simulink model "METI_TRAMI_Thermal_ver01_Jmaab_2018b_Intg"  (R2018b)
settings: Solver=ode8  StartTime=0  StopTime=end_time  FixedStep=sampling_time  RelTol=1e-3
PreLoadFcn:
  | METI_TRAMI_Thermal_ver01_Jmaab_PreLoad;
values from neighbouring files (symbols this model uses):
  degC2K = 273.15    [METI_TRAMI_Thermal_ver01_Jmaab_PreLoad.m]    (also in init_setting_METI.m)
  K2degC = -273.15    [METI_TRAMI_Thermal_ver01_Jmaab_PreLoad.m]    (also in init_setting_METI.m)
undefined symbols (not defined in the file or in its folder): ACC_D_Gain, ACC_I_Gain, ACC_P_Gain, ALT_CNT_ALT_OFF_RPM_HYS_rpm, ALT_CNT_ALT_ON_RPM_HYS_rpm, ALT_CNT_Alter_V_BASE_V, ALT_CNT_Alter_V_Kaisei_V, ALT_CNT_flag_disable_kaisei, ALT_CNT_V_Battely_Kudo_V, ALT_PNT_ALT_GDCurrent_A, ALT_PNT_ALT_GDVolt_V, ALT_PNT_Alter_limit_Current_V_table, ALT_PNT_Alter_limit_Current_V_table_x_rpm, ALT_PNT_Alter_trq_Nm_map, ALT_PNT_Alter_trq_Nm_map_x_rpm, ALT_PNT_Alter_trq_Nm_map_y_Current_A, ALT_PNT_Alter_trq_Nm_map_z_Volt_tgt_V, ALT_PNT_eta_pulley_alt, ALT_PNT_Gain_Alt_v_del, ALT_PNT_ratio_pulley_alt, ALT_PNT_Tau_Alternator_V_tgt_s, ALT_PNT_trq_alter_output_LL_Nm, BK_PNT_Pow_UL, BK_PNT_Tau_brake, Brk_LL, Brk_PGain, Brk_UL, BT_PNT_Lo_Capa_lo_batt_F, BT_PNT_Lo_ocv_SOC_lo_batt_OCV_V_table, BT_PNT_Lo_ocv_SOC_lo_batt_OCV_V_table_x_SOC, BT_PNT_Lo_R_lo_batt_ohm, BT_PNT_Lo_SOC_MAX_lo_batt, BT_PNT_Lo_SOC_MIN_lo_batt, BT_PNT_Lo_SOC_START_lo_batt, BT_PNT_Lo_V_start_ocv, DF_PNT_DF_gear, DF_PNT_DFBlock2DFAir_Heat_Resi_KpW, DF_PNT_DFBlock_Heat_Capa_JpK, DF_PNT_DFBlock_Temp_ini_degC, DF_PNT_DFOil2DFBlock_Heat_Resi_KpW, DF_PNT_DFOil_Heat_Capa_JpK, DF_PNT_DFOil_Temp_ini_degC, DF_PNT_Driveshaft_damper, DF_PNT_Driveshaft_delta_radps_LL, DF_PNT_Driveshaft_delta_radps_UL, DF_PNT_Driveshaft_spring, DF_PNT_eta_DF, DF_PNT_Outtemp_degC, DF_PNT_TMBlock2DFBlock_Heat_Resi_KpW, Driver_Brake_Const1, Driver_Brake_Const3, Driver_Brake_Switch_Const2, Driver_Brk_sh, drivmode_ACC, drivmode_CONST, drivmode_GensokuKaisei, drivmode_GensokuRikko, drivmode_STOP, EL_PNT_R_bodyelec_lo_ohm, ENG_CNT_acc_idlestop ... (+139)
libraries: METI_Lib_vehicle_model x33, simulink x7, AZAPA_Lib_vehicle_model x1
(part 2 of 4)

== system METI_TRAMI_Thermal_ver01_Jmaab_2018b_Intg/Vehicle/ALT_PNT/pulley_slave ==
  note: プーリー比
  note: プーリー効率
  w_ENG_PNT_radps : Inport
  trq_slavepulley12 : Inport  Port=2
  P_cal : AZAPA_Lib_vehicle_model/P_cal  Commented=on  Type_energy=並進運動  Type_output_energy=出力  Power_name=Po_  t_Workspace_Name=MOTOR_MECK  P_VariableName=Po_MOTOR_MECK  Across_VariableName=v_MOTOR_MECK  Throgh_VariableName=F_MOTOR_MECK
  Product : Product  RndMeth=Zero
  Product1 : Product  RndMeth=Zero
  eta_cal2 : METI_Lib_vehicle_model/eta_cal2  SystemSampleTime=-1
  eta_pulley : Constant  Value=ALT_PNT_eta_pulley_alt
  ratio_pulley : Constant  Value=ALT_PNT_ratio_pulley_alt
  trq_slavepulley11 : Outport
  w_slavepulley12 : Outport  Port=2
  tag scope: tScope_pulley1Loss=global
  wires:
  eta_cal2/1 -> P_cal/2
  P_cal/1 -> [tScope_pulley1Loss]
  w_ENG_PNT_radps/1 -> P_cal/1, Product1/1
  eta_cal2/2 -> trq_slavepulley11/1
  trq_slavepulley12/1 -> Product/2
  eta_pulley/1 -> eta_cal2/1
  Product1/1 -> w_slavepulley12/1
  ratio_pulley/1 -> Product/1, Product1/2
  Product/1 -> eta_cal2/2

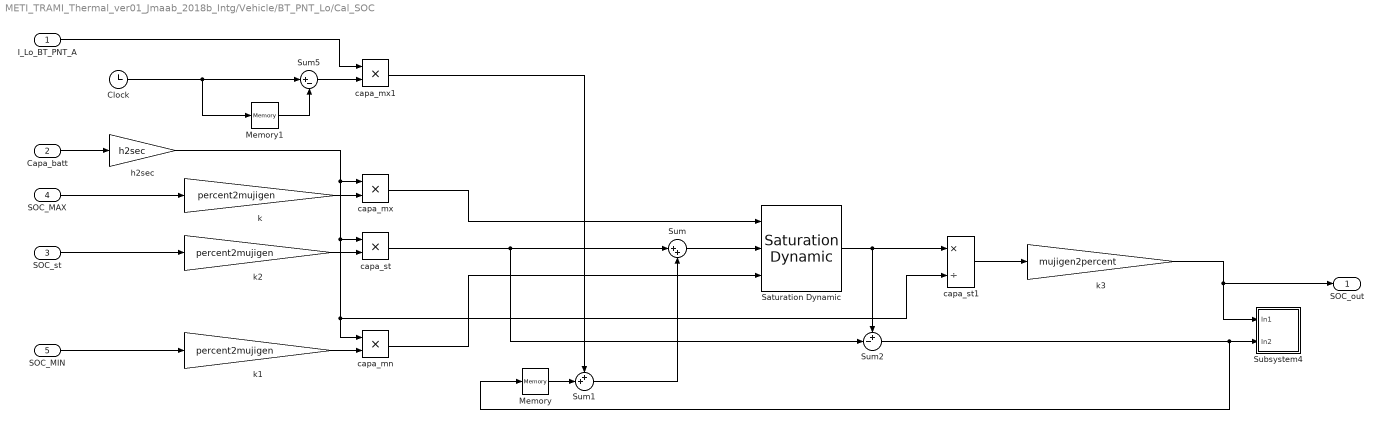
== system METI_TRAMI_Thermal_ver01_Jmaab_2018b_Intg/Vehicle/BT_PNT_Lo/Cal_SOC ==
  I_Lo_BT_PNT_A : Inport
  Capa_batt : Inport  Port=2
  SOC_st : Inport  Port=3
  SOC_MAX : Inport  Port=4
  SOC_MIN : Inport  Port=5
  Clock : Clock
  Memory : Memory
  Memory1 : Memory
  Saturation Dynamic : simulink/Discontinuities/Saturation Dynamic  OutMin=[]  OutMax=[]  OutDataTypeStr=Inherit: Same as second input  OutDataType=fixdt(1, 16)  OutScaling=2^-10  DoSatur=off
  Subsystem4 : Subsystem  mask{SOC=SOC_LoBat, VariableName=Asec_LoBat}
      mask prompts: SOC "バッテリSOC"; VariableName "バッテリ容量変化量(Asec)"
  Sum : Sum  Inputs=|++
  Sum1 : Sum  Inputs=++|
  Sum2 : Sum  Inputs=+-|
  Sum5 : Sum  Inputs=|+-
  capa_mn : Product  RndMeth=Zero
  capa_mx : Product  RndMeth=Zero
  capa_mx1 : Product  RndMeth=Zero
  capa_st : Product  RndMeth=Zero
  capa_st1 : Product  Inputs=*/  RndMeth=Zero
  h2sec : Gain  Gain=h2sec
  k : Gain  Gain=percent2mujigen
  k1 : Gain  Gain=percent2mujigen
  k2 : Gain  Gain=percent2mujigen
  k3 : Gain  Gain=mujigen2percent
  SOC_out : Outport
  wires:
  Sum5/1 -> capa_mx1/2
  Memory1/1 -> Sum5/2
  Sum/1 -> Saturation Dynamic/2
  Clock/1 -> Sum5/1, Memory1/1
  capa_mx1/1 -> Sum1/1
  k3/1 -> Subsystem4/1(In1), SOC_out/1
  Sum1/1 -> Sum/2
  Memory/1 -> Sum1/2
  k2/1 -> capa_st/2
  k1/1 -> capa_mn/2
  k/1 -> capa_mx/2
  capa_st/1 -> Sum2/2, Sum/1
  Saturation Dynamic/1 -> Sum2/1, capa_st1/1
  capa_mx/1 -> Saturation Dynamic/1
  capa_mn/1 -> Saturation Dynamic/3
  capa_st1/1 -> k3/1
  h2sec/1 -> capa_mn/1, capa_st1/2, capa_st/1, capa_mx/1
  SOC_MIN/1 -> k1/1
  SOC_MAX/1 -> k/1
  SOC_st/1 -> k2/1
  Capa_batt/1 -> h2sec/1
  I_Lo_BT_PNT_A/1 -> capa_mx1/1
  Sum2/1 -> Memory/1, Subsystem4/2(In2)

== system METI_TRAMI_Thermal_ver01_Jmaab_2018b_Intg/Vehicle/BT_PNT_Lo/Subsystem ==
  I_BT_PNT_Lo_A : Inport
  Divide : Product
  Resistivity : Constant  Value=BT_PNT_Lo_R_lo_batt_ohm
  Sum : Sum  Inputs=|++
  Transfer Fcn : TransferFcn  Numerator=[0.01]  Denominator=[0.1 1]
  V_BT_PNT_Lo_V : Outport
  wires:
  Resistivity/1 -> Divide/2
  Divide/1 -> Sum/1
  I_BT_PNT_Lo_A/1 -> Divide/1, Transfer Fcn/1
  Sum/1 -> V_BT_PNT_Lo_V/1
  Transfer Fcn/1 -> Sum/2

== system METI_TRAMI_Thermal_ver01_Jmaab_2018b_Intg/Vehicle/CNT/ALT_CNT ==
  sensor_BT_PNT_Lo_BUS : Inport
  ALT_Ctrl : Subsystem
  Bus Creator6 : BusCreator  Inputs=1
  Bus Selector1 : BusSelector  OutputSignals=flag_fuelcut,flag_IdleStop,n_eng_rpm
  Bus Selector9 : BusSelector  OutputSignals=SOC_BT_PNT_Lo_PCT
  ALT_CNT_out : Outport
  wires:
  [ALT_CNT_CAN_Rx] -> Bus Selector1/1
  Bus Selector1/1 -> ALT_Ctrl/2(flag_fuelcut)  "<flag_fuelcut>"
  Bus Selector1/2 -> ALT_Ctrl/3(flag_IdleStop)  "<flag_IdleStop>"
  Bus Selector1/3 -> ALT_Ctrl/4(n_eng_rpm)  "<n_eng_rpm>"
  ALT_Ctrl/1(target_volt_ALT_V) -> Bus Creator6/1
  sensor_BT_PNT_Lo_BUS/1 -> Bus Selector9/1
  Bus Selector9/1 -> ALT_Ctrl/1(SOC_BT_PNT_Lo_PCT)  "<SOC_BT_PNT_Lo_PCT>"
  Bus Creator6/1 -> ALT_CNT_out/1  "ALT_CNT_out"

== system METI_TRAMI_Thermal_ver01_Jmaab_2018b_Intg/Vehicle/CNT/BK_CNT ==
  Driver_Input : Inport
  sensor_VL_PNT_BUS : Inport  Port=2
  sensor_BK_PNT : Inport  Port=3
  BK_Ctrl : Subsystem
  Bus Creator1 : BusCreator  Inputs=1
  Bus Creator2 : BusCreator  Inputs=2
  Bus Selector1 : BusSelector  OutputSignals=trq_BK_PNT_Nm
  Bus Selector12 : BusSelector  OutputSignals=v_VL_PNT_kmph
  Bus Selector4 : BusSelector  OutputSignals=open_brake_per
  BK_CNT_out : Outport
  tag scope: BK_CNT_CAN_Tx=scoped
  wires:
  BK_Ctrl/2(v_VL_PNT_kmph) -> Bus Creator2/1
  Bus Selector12/1 -> BK_Ctrl/2(v_VL_PNT_kmph_in)  "<v_VL_PNT_kmph>"
  sensor_VL_PNT_BUS/1 -> Bus Selector12/1
  BK_Ctrl/3(trq_BK_PNT_Nm) -> Bus Creator2/2
  Bus Creator2/1 -> [BK_CNT_CAN_Tx]  "BK_CNT_CAN_Tx"
  Bus Selector1/1 -> BK_Ctrl/3(trq_BK_PNT_Nm_in)  "<trq_BK_PNT_Nm>"
  sensor_BK_PNT/1 -> Bus Selector1/1
  Bus Creator1/1 -> BK_CNT_out/1  "BK_CNT_out"
  Bus Selector4/1 -> BK_Ctrl/1(open_brake_per_in)  "<open_brake_per>"
  Driver_Input/1 -> Bus Selector4/1
  BK_Ctrl/1(open_brake_per) -> Bus Creator1/1

== system METI_TRAMI_Thermal_ver01_Jmaab_2018b_Intg/Vehicle/CNT/CAN ==
  note: CAN Bus Model
  ALT_CNT : Subsystem
  BK_CNT : Subsystem
  ENG_CNT : Subsystem
  Pwtr_CAN : Subsystem
  TM_CNT : Subsystem
  wires:
  Pwtr_CAN/1(Pwtr_CAN) -> BK_CNT/1(Pwtr_CAN), ALT_CNT/1(Pwtr_CAN), TM_CNT/1(Pwtr_CAN), ENG_CNT/1(Pwtr_CAN)
  ENG_CNT/1(ENG_CNT_CAN_Tx) -> Pwtr_CAN/1(ENG_CNT_CAN_Tx)
  TM_CNT/1(TM_CNT_CAN_Tx) -> Pwtr_CAN/2(TM_CNT_CAN_Tx)
  BK_CNT/1(BK_CNT_CAN_Tx) -> Pwtr_CAN/3(BK_CNT_CAN_Tx)

== system METI_TRAMI_Thermal_ver01_Jmaab_2018b_Intg/Vehicle/CNT/ENG_CNT ==
  Driver_Input : Inport
  sensor_ENG_PNT : Inport  Port=2
  Bus Creator : BusCreator  Inputs=6
  Bus Creator1 : BusCreator  Inputs=10
  Bus Selector1 : BusSelector  OutputSignals=v_VL_PNT_kmph,flag_Lockup
  Bus Selector13 : BusSelector  OutputSignals=n_eng_rpm,fuel_consumption,T_ENGTH_PNT_Coolant_degC
  Bus Selector14 : BusSelector  OutputSignals=open_accel_per,open_brake_per
  ENG_Cntrl : Subsystem
  ENG_CNT_out : Outport
  tag scope: ENG_CNT_CAN_Tx=scoped
  wires:
  ENG_Cntrl/11(IdleSpeed_Target) -> Bus Creator/5
  Bus Selector1/1 -> ENG_Cntrl/6(v_VL_PNT_kmph)  "<v_VL_PNT_kmph>"
  Bus Selector13/3 -> ENG_Cntrl/5(T_ENGTH_PNT_Coolant_degC), Bus Creator/6  "<T_ENGTH_PNT_Coolant_degC>"
  Bus Selector13/2 -> ENG_Cntrl/4(fuel_consumption)  "<fuel_consumption>"
  ENG_Cntrl/10(V_ENG_CNT_RDFan_V) -> Bus Creator1/10
  ENG_Cntrl/9(V_ENG_CNT_WP_V) -> Bus Creator1/9
  ENG_Cntrl/8(K_Fuel) -> Bus Creator1/8
  Bus Selector1/2 -> ENG_Cntrl/7(flag_Lockup)  "<flag_Lockup>"
  [ENG_CNT_CAN_Rx] -> Bus Selector1/1
  Bus Selector14/2 -> ENG_Cntrl/2(open_brake_per)  "<open_brake_per>"
  Bus Selector14/1 -> ENG_Cntrl/1(open_accel_per)  "<open_accel_per>"
  Driver_Input/1 -> Bus Selector14/1
  Bus Selector13/1 -> ENG_Cntrl/3(sens_ENG_PNT)  "<n_eng_rpm>"
  sensor_ENG_PNT/1 -> Bus Selector13/1
  Bus Creator1/1 -> ENG_CNT_out/1  "ENG_CNT_out"
  ENG_Cntrl/7(flag_ON_Starter) -> Bus Creator1/7
  ENG_Cntrl/6(n_eng_rpm) -> Bus Creator1/6, Bus Creator/4
  ENG_Cntrl/5(timing_ignition) -> Bus Creator1/5
  ENG_Cntrl/4(fuel_ratio) -> Bus Creator1/4
  ENG_Cntrl/3(flag_fuelcut) -> Bus Creator1/3, Bus Creator/3
  ENG_Cntrl/2(flag_IdleStop) -> Bus Creator1/2, Bus Creator/2
  ENG_Cntrl/1(open_throttle_per) -> Bus Creator1/1, Bus Creator/1
  Bus Creator/1 -> [ENG_CNT_CAN_Tx]  "ENG_CNT_CAN_Tx"

== system METI_TRAMI_Thermal_ver01_Jmaab_2018b_Intg/Vehicle/CNT/TM_CNT ==
  sensor_TM_PNT : Inport
  Rate Transition : RateTransition  Deterministic=off
      settings: AttributesFormatString=|
      | <Integrity = %<Integrity>>
      | <Deterministic = %<Deterministic>>
  Rate Transition1 : RateTransition  Deterministic=off
      settings: AttributesFormatString=|
      | <Integrity = %<Integrity>>
      | <Deterministic = %<Deterministic>>
  Rate Transition2 : RateTransition  Deterministic=off
      settings: AttributesFormatString=|
      | <Integrity = %<Integrity>>
      | <Deterministic = %<Deterministic>>
  TM_CNT : Subsystem  Variant=on  VariantControl=Variant1
  TM_CNT_out : Outport
  tag scope: TM_CNT_CAN_Tx=scoped, TM_CNT_Info=global
  wires:
  sensor_TM_PNT/1 -> Rate Transition/1
  [TM_CNT_CAN_Rx] -> Rate Transition1/1
  Rate Transition2/1 -> TM_CNT_out/1  "TM_CNT_out"
  Rate Transition/1 -> TM_CNT/1("sensor_TM_PNT ")
  Rate Transition1/1 -> TM_CNT/2("TM_CNT_CAN_Rx ")
  TM_CNT/1(" TM_CNT_out") -> Rate Transition2/1
  TM_CNT/2(" TM_CNT_CAN_Tx") -> [TM_CNT_CAN_Tx]
  TM_CNT/3(" TM_CNT_Info") -> [TM_CNT_Info]

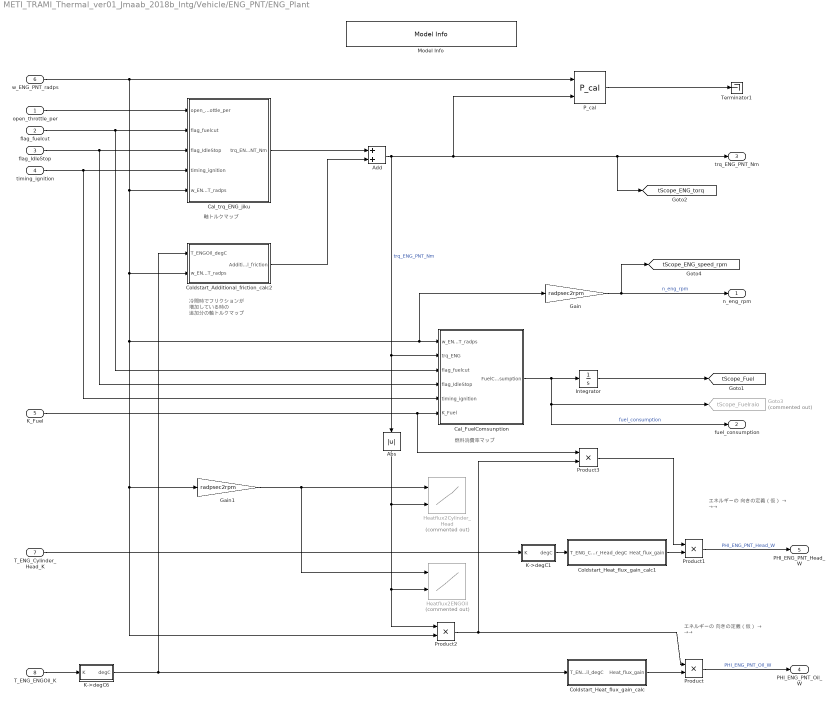
== system METI_TRAMI_Thermal_ver01_Jmaab_2018b_Intg/Vehicle/ENG_PNT/ENG_Plant ==
  note: 軸トルクマップ
  note: 燃料消費率マップ
  note: 冷間時でフリクションが
      | 増加している時の
      | 追加分の軸トルクマップ
  note: エネルギーの
      | 向きの定義（仮）
      | → →→
  note: エネルギーの
      | 向きの定義（仮）
      | → →→
  open_throttle_per : Inport
  flag_fuelcut : Inport  Port=2
  flag_IdleStop : Inport  Port=3
  timing_ignition : Inport  Port=4
  K_Fuel : Inport  Port=5
  w_ENG_PNT_radps : Inport  Port=6
  T_ENG_Cylinder_Head_K : Inport  Port=7
  T_ENG_ENGOil_K : Inport  Port=8
  Abs : Abs
  Add : Sum
  Cal_FuelComsunption : Subsystem
  Cal_trq_ENG_jiku : Subsystem
  Coldstart_Additional_friction_calc2 : Subsystem
  Coldstart_Heat_flux_gain_calc : Subsystem
  Coldstart_Heat_flux_gain_calc1 : Subsystem
  Gain : Gain  Gain=radpsec2rpm
  Gain1 : Gain  Gain=radpsec2rpm
  Goto3 : Goto  Commented=on  GotoTag=tScope_Fuelraio  TagVisibility=global
  Heatflux2Cylinder_Head : Lookup_n-D  Commented=on  BreakpointsForDimension1=ENG_PNT_Heatflux2Cylinder_Head_W_x_rpm  BreakpointsForDimension2=ENG_PNT_Heatflux2Cylinder_Head_W_y_trq  Table=ENG_PNT_Heatflux2Cylinder_Head_W  InternalRulePriority=Speed  RndMeth=Simplest  InputSameDT=on
  Heatflux2ENGOil : Lookup_n-D  Commented=on  BreakpointsForDimension1=ENG_PNT_Heatflux2ENGOil_W_x_rpm  BreakpointsForDimension2=ENG_PNT_Heatflux2ENGOil_W_y_trq  Table=ENG_PNT_Heatflux2ENGOil_W  InternalRulePriority=Speed  RndMeth=Simplest  InputSameDT=on
  Integrator : Integrator
  K->degC1 : Subsystem
  K->degC6 : Subsystem
  Model Info : simulink/Model-Wide Utilities/Model Info  Frame=on  DisplayStringWithTags=【注記】 ・エンジンモデルはトルク出力動作させる側が正  HorizontalTextAlignment=Left  LeftAlignmentValue=0.02
  P_cal : METI_Lib_vehicle_model/P_cal  Type_energy=回転運動  Type_output_energy=出力  Power_name=Po_  t_Workspace_Name=ENG_PNT_MECK  P_VariableName=Po_ENG_PNT_MECK  Across_VariableName=w_ENG_PNT_MECK  Throgh_VariableName=tq_ENG_PNT_MECK
  Product{,1..3} (4 alike) : Product
  Terminator1 : Terminator
  n_eng_rpm : Outport
  fuel_consumption : Outport  Port=2
  trq_ENG_PNT_Nm : Outport  Port=3
  PHI_ENG_PNT_Oil_W : Outport  Port=4
  PHI_ENG_PNT_Head_W : Outport  Port=5
  tag scope: tScope_ENG_speed_rpm=global, tScope_ENG_torq=global, tScope_Fuel=global
  wires:
  Cal_FuelComsunption/1(FuelConsumption) -> fuel_consumption/1, Goto3/1, Integrator/1  "fuel_consumption"
  Integrator/1 -> [tScope_Fuel]
  w_ENG_PNT_radps/1 -> P_cal/1, Coldstart_Additional_friction_calc2/2(w_ENG_PNT_radps), Gain1/1, Product2/2, Gain/1, Cal_FuelComsunption/1(w_ENG_PNT_radps), Cal_trq_ENG_jiku/5(w_ENG_PNT_radps)
  P_cal/1 -> Terminator1/1
  flag_fuelcut/1 -> Cal_trq_ENG_jiku/2(flag_fuelcut), Cal_FuelComsunption/3(flag_fuelcut)
  flag_IdleStop/1 -> Cal_FuelComsunption/4(flag_IdleStop), Cal_trq_ENG_jiku/3(flag_IdleStop)
  open_throttle_per/1 -> Cal_trq_ENG_jiku/1(open_throttle_per)
  Cal_trq_ENG_jiku/1(trq_ENG_PNT_Nm) -> Add/1
  timing_ignition/1 -> Cal_FuelComsunption/5(timing_ignition), Cal_trq_ENG_jiku/4(timing_ignition)
  Gain/1 -> [tScope_ENG_speed_rpm], n_eng_rpm/1  "n_eng_rpm"
  K->degC6/1(degC) -> Coldstart_Heat_flux_gain_calc/1(T_ENGOil_degC), Coldstart_Additional_friction_calc2/1(T_ENGOil_degC)
  T_ENG_Cylinder_Head_K/1 -> K->degC1/1(K)
  Product1/1 -> PHI_ENG_PNT_Head_W/1  "PHI_ENG_PNT_Head_W"
  Product/1 -> PHI_ENG_PNT_Oil_W/1  "PHI_ENG_PNT_Oil_W"
  Gain1/1 -> Heatflux2ENGOil/1, Heatflux2Cylinder_Head/1
  Coldstart_Heat_flux_gain_calc/1(Heat_flux_gain) -> Product/2
  Product2/1 -> Product/1, Product3/2
  Coldstart_Heat_flux_gain_calc1/1(Heat_flux_gain) -> Product1/2
  Coldstart_Additional_friction_calc2/1(Additional_friction) -> Add/2
  Add/1 -> [tScope_ENG_torq], trq_ENG_PNT_Nm/1, P_cal/2, Cal_FuelComsunption/2(trq_ENG), Abs/1  "trq_ENG_PNT_Nm"
  K_Fuel/1 -> Product3/1, Cal_FuelComsunption/6(K_Fuel)
  Abs/1 -> Product2/1, Heatflux2ENGOil/2, Heatflux2Cylinder_Head/2
  Product3/1 -> Product1/1
  T_ENG_ENGOil_K/1 -> K->degC6/1(K)
  K->degC1/1(degC) -> Coldstart_Heat_flux_gain_calc1/1(T_ENG_Cylinder_Head_degC)

== system METI_TRAMI_Thermal_ver01_Jmaab_2018b_Intg/Vehicle/ENG_PNT/K->degC ==
  K : Inport
  Constant2 : Constant  Value=K2degC
  Sum : Sum  Inputs=++|
  degC : Outport
  wires:
  K/1 -> Sum/2
  Constant2/1 -> Sum/1
  Sum/1 -> degC/1

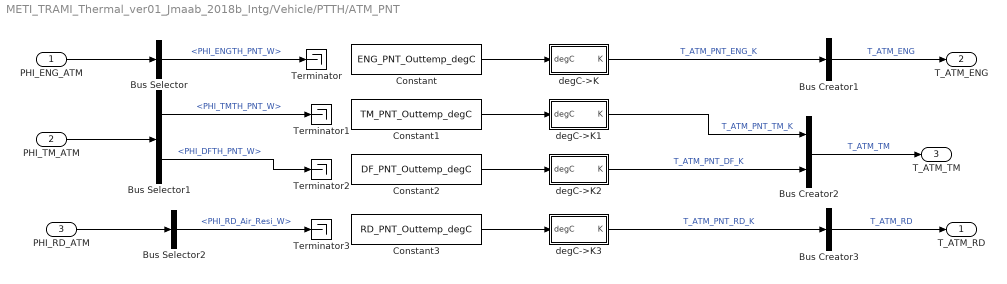
== system METI_TRAMI_Thermal_ver01_Jmaab_2018b_Intg/Vehicle/PTTH/ATM_PNT ==
  PHI_ENG_ATM : Inport
  PHI_TM_ATM : Inport  Port=2
  PHI_RD_ATM : Inport  Port=3
  Bus Creator1 : BusCreator  Inputs=1
  Bus Creator2 : BusCreator  Inputs=2
  Bus Creator3 : BusCreator  Inputs=1
  Bus Selector : BusSelector  OutputSignals=PHI_ENGTH_PNT_W
  Bus Selector1 : BusSelector  OutputSignals=PHI_TMTH_PNT_W,PHI_DFTH_PNT_W
  Bus Selector2 : BusSelector  OutputSignals=PHI_RD_Air_Resi_W
  Constant : Constant  Value=ENG_PNT_Outtemp_degC
  Constant1 : Constant  Value=TM_PNT_Outtemp_degC
  Constant2 : Constant  Value=DF_PNT_Outtemp_degC
  Constant3 : Constant  Value=RD_PNT_Outtemp_degC
  Terminator{,1..3} (4 alike) : Terminator
  degC->K : Subsystem
  degC->K1 : Subsystem
  degC->K2 : Subsystem
  degC->K3 : Subsystem
  T_ATM_RD : Outport
  T_ATM_ENG : Outport  Port=2
  T_ATM_TM : Outport  Port=3
  wires:
  Constant/1 -> degC->K/1(degC)
  Constant1/1 -> degC->K1/1(degC)
  Constant2/1 -> degC->K2/1(degC)
  Constant3/1 -> degC->K3/1(degC)
  Bus Selector1/2 -> Terminator2/1  "<PHI_DFTH_PNT_W>"
  degC->K/1(K) -> Bus Creator1/1  "T_ATM_PNT_ENG_K"
  degC->K1/1(K) -> Bus Creator2/1  "T_ATM_PNT_TM_K"
  degC->K2/1(K) -> Bus Creator2/2  "T_ATM_PNT_DF_K"
  degC->K3/1(K) -> Bus Creator3/1  "T_ATM_PNT_RD_K"
  PHI_ENG_ATM/1 -> Bus Selector/1
  Bus Selector/1 -> Terminator/1  "<PHI_ENGTH_PNT_W>"
  PHI_TM_ATM/1 -> Bus Selector1/1
  Bus Selector1/1 -> Terminator1/1  "<PHI_TMTH_PNT_W>"
  Bus Creator2/1 -> T_ATM_TM/1  "T_ATM_TM"
  Bus Creator1/1 -> T_ATM_ENG/1  "T_ATM_ENG"
  Bus Creator3/1 -> T_ATM_RD/1  "T_ATM_RD"
  PHI_RD_ATM/1 -> Bus Selector2/1
  Bus Selector2/1 -> Terminator3/1  "<PHI_RD_Air_Resi_W>"

== system METI_TRAMI_Thermal_ver01_Jmaab_2018b_Intg/Vehicle/PTTH/DTTH_PNT ==
  T_ENG_TM : Inport
  TM_CNT_out : Inport  Port=2
  PHI_TM_PNT : Inport  Port=3
  v_VL_PNT_mps : Inport  Port=4
  T_RD_TM : Inport  Port=5
  T_ATM_TM : Inport  Port=6
  DTTH_PNT : Subsystem  Variant=on  VariantControl=Variant1
  Memory1 : Memory
  T_TMTH_PNT : Outport
  PHI_TM_ATM : Outport  Port=2
  PHI_TM_RD : Outport  Port=3
  PHI_TM_ENG : Outport  Port=4
  tag scope: TMTH_Info=global
  wires:
  Memory1/1 -> T_TMTH_PNT/1  "T_TMTH_PNT"
  TM_CNT_out/1 -> DTTH_PNT/1("TM_CNT_out ")
  PHI_TM_PNT/1 -> DTTH_PNT/2("PHI_TM_PNT ")
  T_ENG_TM/1 -> DTTH_PNT/3("T_ENG_TM ")
  T_RD_TM/1 -> DTTH_PNT/4("T_RD_TM ")
  T_ATM_TM/1 -> DTTH_PNT/5("T_ATM_TM ")
  v_VL_PNT_mps/1 -> DTTH_PNT/6("v_VL_PNT_mps ")
  DTTH_PNT/1(" T_TMTH_PNT") -> Memory1/1
  DTTH_PNT/2(" PHI_TM_ENG") -> PHI_TM_ENG/1
  DTTH_PNT/3(" PHI_TM_RD") -> PHI_TM_RD/1
  DTTH_PNT/4(" PHI_TM_ATM") -> PHI_TM_ATM/1
  DTTH_PNT/5(" TMTH_Info") -> [TMTH_Info]

== system METI_TRAMI_Thermal_ver01_Jmaab_2018b_Intg/Vehicle/PTTH/ENGTH_PNT ==
  ENG_CNT_out : Inport
  PHI_ENG_PNT : Inport  Port=2
  PHI_RD_ENG : Inport  Port=3
  T_ATM_ENG : Inport  Port=4
  PHI_TM_ENG : Inport  Port=5
  Bus Creator1 : BusCreator  Inputs=3
  Bus Creator2 : BusCreator  Inputs=2
  Bus Creator3 : BusCreator  Inputs=4
  Bus Creator4 : BusCreator  Inputs=1
  Bus Creator5 : BusCreator  Inputs=1
  Bus Selector : BusSelector  OutputSignals=V_ENG_CNT_WP_V
  Bus Selector1 : BusSelector  OutputSignals=PHI_ENG_PNT_Head_W,PHI_ENG_PNT_Oil_W
  Bus Selector2 : BusSelector  OutputSignals=PHI_ENGBlock_Resi2_W,PHI_TM_CVTF_Resi_W
  Bus Selector3 : BusSelector  OutputSignals=T_ATM_PNT_ENG_K
  Bus Selector4 : BusSelector  OutputSignals=PHI_RDTH_PNT_W
  ENGTH : Subsystem
  Signal Specification2 : SignalSpecification
  Signal Specification3 : SignalSpecification
  T_ENGTH_PNT : Outport
  PHI_ENG_ATM : Outport  Port=2
  T_ENG_TM : Outport  Port=3
  T_ENG_RD : Outport  Port=4
  tag scope: ENGTH_Info=global
  wires:
  ENG_CNT_out/1 -> Bus Selector/1
  ENGTH/1(T_ENGTH_PNT_Coolant_K) -> Bus Creator3/4, Bus Creator1/2, Bus Creator2/1, Bus Creator4/1
  ENGTH/2(T_ENG_Block_K) -> Bus Creator3/1, Bus Creator2/2
  ENGTH/3(T_ENGTH_PNT_Oil_K) -> Bus Creator3/2, Signal Specification3/1
  ENGTH/4(T_ENGTH_PNT_Head_K) -> Bus Creator3/3, Signal Specification2/1
  ENGTH/5(PHI_ENGTH_PNT_W) -> Bus Creator5/1
  Bus Selector/1 -> ENGTH/1(V_ENG_CNT_WP_V)  "<V_ENG_CNT_WP_V>"
  PHI_ENG_PNT/1 -> Bus Selector1/1
  Bus Selector1/1 -> ENGTH/3(PHI_ENG_PNT_Head_W)  "<PHI_ENG_PNT_Head_W>"
  Bus Selector1/2 -> ENGTH/4(PHI_ENG_PNT_Oil_W)  "<PHI_ENG_PNT_Oil_W>"
  Bus Creator1/1 -> T_ENGTH_PNT/1  "T_ENGTH_PNT"
  Signal Specification2/1 -> Bus Creator1/1  "T_ENGTH_PNT__Head_K"
  Signal Specification3/1 -> Bus Creator1/3  "T_ENGTH_PNT_Oil_K"
  Bus Creator2/1 -> T_ENG_TM/1  "T_ENG_TM"
  Bus Creator4/1 -> T_ENG_RD/1  "T_ENG_RD"
  Bus Creator5/1 -> PHI_ENG_ATM/1  "PHI_ENG_ATM"
  Bus Creator3/1 -> [ENGTH_Info]  "ENGTH_Info"
  PHI_TM_ENG/1 -> Bus Selector2/1
  Bus Selector2/1 -> ENGTH/2(PHI_ENGBlock_W)  "<PHI_ENGBlock_Resi2_W>"
  Bus Selector2/2 -> ENGTH/6(PHI_TM_CVTF_Resi_W)  "<PHI_TM_CVTF_Resi_W>"
  T_ATM_ENG/1 -> Bus Selector3/1
  PHI_RD_ENG/1 -> Bus Selector4/1
  Bus Selector3/1 -> ENGTH/5(T_ATM_PNT_ENG_K)  "<T_ATM_PNT_ENG_K>"
  Bus Selector4/1 -> ENGTH/7(PHI_ENGCoolant_W1)  "<PHI_RDTH_PNT_W>"

== system METI_TRAMI_Thermal_ver01_Jmaab_2018b_Intg/Vehicle/PTTH/RDTH_PNT ==
  PHI_TM_RD : Inport
  T_ENG_RD : Inport  Port=2
  ENG_CNT_out : Inport  Port=3
  v_VL_PNT_mps : Inport  Port=4
  T_ATM_RD : Inport  Port=5
  Bus Creator : BusCreator  Inputs=1
  Bus Creator1 : BusCreator  Inputs=1
  Bus Creator2 : BusCreator  Inputs=1
  Bus Creator4 : BusCreator  Inputs=2
  Bus Selector : BusSelector  OutputSignals=V_ENG_CNT_RDFan_V
  Bus Selector1 : BusSelector  OutputSignals=T_ENGTH_PNT_Coolant_K
  Bus Selector2 : BusSelector  OutputSignals=T_ATM_PNT_RD_K
  Bus Selector3 : BusSelector  OutputSignals=PHI_Oil_TM_RD
  RDTH : Subsystem
  Terminator : Terminator
  mps2kmph : Gain  Gain=mps2kmph
  zero : Constant  Value=0
  PHI_RD_ATM : Outport
  PHI_RD_ENG : Outport  Port=2
  T_RD_TM : Outport  Port=3
  tag scope: RDTH_Info=global
  wires:
  v_VL_PNT_mps/1 -> mps2kmph/1
  RDTH/1(T_RDCoolant_degC) -> Bus Creator4/1
  RDTH/2(PHI_RDTH_PNT_W) -> Bus Creator4/2, Bus Creator1/1
  RDTH/3(PHI_RD_Air_Resi_W) -> Bus Creator2/1
  ENG_CNT_out/1 -> Bus Selector/1
  Bus Selector/1 -> RDTH/1(RD_PNT_Voltage_RDFan_V)  "<V_ENG_CNT_RDFan_V>"
  T_ENG_RD/1 -> Bus Selector1/1
  Bus Selector1/1 -> RDTH/3(T_ENGTH_PNT_Coolant_K)  "<T_ENGTH_PNT_Coolant_K>"
  mps2kmph/1 -> RDTH/2(v_VL_PNT_kmph)  "v_VL_PNT_kmph"
  Bus Creator4/1 -> [RDTH_Info]  "RDTH_Info"
  Bus Creator1/1 -> PHI_RD_ENG/1  "PHI_RD_ENG"
  Bus Creator2/1 -> PHI_RD_ATM/1  "PHI_RD_ATM"
  T_ATM_RD/1 -> Bus Selector2/1
  Bus Selector2/1 -> RDTH/4(T_ATM_PNT_RD_K)  "<T_ATM_PNT_RD_K>"
  PHI_TM_RD/1 -> Bus Selector3/1
  Bus Selector3/1 -> Terminator/1  "<PHI_Oil_TM_RD>"
  Bus Creator/1 -> T_RD_TM/1  "T_RD_TM"
  zero/1 -> Bus Creator/1  "T_PT_TH_K"

== system METI_TRAMI_Thermal_ver01_Jmaab_2018b_Intg/Vehicle/TM_PNT/TM_PNT ==
  "TM_CNT_out " : Inport
  "trq_ENG_PNT_Nm " : Inport  Port=2
  "trq_ALT_PNT_Nm " : Inport  Port=3
  "trq__ST_PNT_Nm " : Inport  Port=4
  "w_TR_PNT_radps " : Inport  Port=5
  "T_TMTH_PNT " : Inport  Port=6
  TM_PNT : Subsystem  TreatAsAtomicUnit=on  VariantControl=VarObj_METI_Subsys
      settings: AttributesFormatString="<AtomicUnit =  %<TreatAsAtomicUnit>>"
  TM_PNT1 : ModelReference  ModelNameDialog=METI_TM_PNT  SimulationMode=Normal  VariantControl=VarObj_METI_Mref  ModelReferenceVersion=1.420
  TM_PNT2 : ModelReference  ModelNameDialog=TRAMI_TM_PNT.slx  SimulationMode=Normal  VariantControl=VarObj_TRAMI_Mref  ModelReferenceVersion=1.399
  " sensor_TM_PNT" : Outport
  " trq_DS_PNT_Nm" : Outport  Port=2
  " w_ENG_PNT_radps" : Outport  Port=3
  " PHI_TM_PNT" : Outport  Port=4
  " TM_PNT_Info" : Outport  Port=5

== system METI_TRAMI_Thermal_ver01_Jmaab_2018b_Intg/Driver/Driver/Driver/Caliculate_Driving_State ==
  open_brake_per : Inport
  target_v_VL_kmph : Inport  Port=2
  Constant : Constant  Value=Thresh_Stop_vCar
  Constant4 : Constant  Value=0.1*sampling_time
  Constant6 : Constant  Value=-0.1*sampling_time
  Memory : Memory
  Relational Operator : RelationalOperator  Operator=>  OutDataTypeStr=boolean  RndMeth=Nearest
  Relational Operator1 : RelationalOperator  Operator=<  OutDataTypeStr=boolean  RndMeth=Nearest
  Relational Operator2 : RelationalOperator  Operator=<  OutDataTypeStr=boolean  RndMeth=Nearest
  Sum : Sum  Inputs=|+-
  Switch{,1..3} (4 alike) : Switch  Criteria=u2 > Threshold  Threshold=0.5
  Terminator : Terminator
  停止 : Constant  Value=drivmode_STOP
  加速 : Constant  Value=drivmode_ACC
  定常1 : Constant  Value=drivmode_CONST
  減速力行 : Constant  Value=drivmode_GensokuRikko
  減速回生 : Constant  Value=drivmode_GensokuKaisei
  wires:
  Switch/1 -> Terminator/1  "state_driving"
  target_v_VL_kmph/1 -> Relational Operator/1, Memory/1, Sum/1
  Relational Operator1/1 -> Switch1/2
  Constant4/1 -> Relational Operator1/2
  Relational Operator/1 -> Switch/2
  Constant/1 -> Relational Operator/2
  停止/1 -> Switch/3
  Sum/1 -> Relational Operator1/1, Relational Operator2/1
  減速回生/1 -> Switch2/1
  Switch3/1 -> Switch1/1
  Constant6/1 -> Relational Operator2/2
  Memory/1 -> Sum/2
  open_brake_per/1 -> Switch2/2
  減速力行/1 -> Switch2/3
  Relational Operator2/1 -> Switch3/2
  Switch2/1 -> Switch3/1
  定常1/1 -> Switch3/3
  加速/1 -> Switch1/3
  Switch1/1 -> Switch/1

== system METI_TRAMI_Thermal_ver01_Jmaab_2018b_Intg/Driver/Driver/Driver/Caliculate_Opeining_Accel ==
  v_VL_PNT_kmph : Inport
  target_v_VL_kmph : Inport  Port=2
  pre_n_eng_rpm : Inport  Port=3
  pre_ratio_CVT : Inport  Port=4
  FB : Subsystem  mask{P_Gain=ACC_P_Gain, D_Gain=ACC_D_Gain, I_Gain=ACC_I_Gain}
      mask prompts: P_Gain "Pゲイン値"; D_Gain "Dゲイン値"; I_Gain "Iゲイン値"
  FF : Subsystem
  Guard_0_100 : Saturate  UpperLimit=ENG_CNT_Throttle_UL  LowerLimit=ENG_CNT_Throttle_LL
  Sum1 : Sum  Inputs=|-+
  Sum3 : Sum  Inputs=++|
  open_accel_per : Outport
  wires:
  Sum1/1 -> FB/1(delta_v_VL_kmph)
  v_VL_PNT_kmph/1 -> FF/1(v_VL_PNT_kmph), Sum1/1
  target_v_VL_kmph/1 -> FF/2(target_v_VL_kmph), Sum1/2
  Sum3/1 -> Guard_0_100/1
  pre_n_eng_rpm/1 -> FF/3(pre_n_eng_rpm)
  pre_ratio_CVT/1 -> FF/4(pre_ratio_CVT)
  FB/1(FB_open_accel_per) -> Sum3/1
  FF/1(FF_open_accel_per) -> Sum3/2
  Guard_0_100/1 -> open_accel_per/1  "open_accel_per"

== system METI_TRAMI_Thermal_ver01_Jmaab_2018b_Intg/Driver/Driver/Driver/Caliculate_Opening_Brake ==
  v_VL_PNT_kmph : Inport
  target_v_VL_kmph : Inport  Port=2
  open_accel_per : Inport  Port=3
  Constant : Constant  Value=Driver_Brake_Const1
  Constant1 : Constant  Value=Driver_Brk_sh
  Constant2 : Constant  Value=Driver_Brake_Const3
  Constant3 : Constant  Value=0
  F2per : Gain  Gain=1/Brk_UL*100
  Logical Operator : Logic  AllPortsSameDT=off  OutDataTypeStr=boolean
  Memory : Memory
  Memory1 : Memory
  PGain : Gain  Gain=Brk_PGain
  PGain1 : Gain  Gain=Brk_PGain
  Relational Operator : RelationalOperator  OutDataTypeStr=boolean  RndMeth=Nearest
  Relational Operator1 : RelationalOperator  Operator=>  OutDataTypeStr=boolean  RndMeth=Nearest
  Saturation : Saturate  UpperLimit=Brk_UL  LowerLimit=Brk_LL
  Sum1 : Sum  Inputs=|-+
  Sum2 : Sum  Inputs=|+-
  Switch : Switch  Threshold=0.5
  Switch1 : Switch  Criteria=u2 > Threshold  Threshold=Driver_Brake_Switch_Const2
  open_brake_per : Outport
  wires:
  target_v_VL_kmph/1 -> Switch1/2, Sum1/2, Memory1/1, Sum2/1
  Sum1/1 -> PGain/1
  PGain/1 -> Saturation/1
  Constant/1 -> PGain1/1
  PGain1/1 -> Switch1/3
  open_accel_per/1 -> Memory/1
  Memory/1 -> Relational Operator1/1
  Memory1/1 -> Sum2/2
  Switch/1 -> F2per/1
  Sum2/1 -> Relational Operator/1
  Saturation/1 -> Switch1/1
  Switch1/1 -> Switch/3
  Constant2/1 -> Switch/1
  v_VL_PNT_kmph/1 -> Sum1/1
  Constant1/1 -> Relational Operator/2
  Constant3/1 -> Relational Operator1/2
  Relational Operator1/1 -> Logical Operator/2
  Relational Operator/1 -> Logical Operator/1
  Logical Operator/1 -> Switch/2
  F2per/1 -> open_brake_per/1  "open_brake_per"

== system METI_TRAMI_Thermal_ver01_Jmaab_2018b_Intg/Driver/Driver_TRAMI/Driver2/Caliculate_Driving_State ==
  open_brake_per : Inport
  target_v_VL_kmph : Inport  Port=2
  Constant : Constant  Value=Thresh_Stop_vCar
  Constant4 : Constant  Value=0.1*sampling_time
  Constant6 : Constant  Value=-0.1*sampling_time
  Memory : Memory
  Relational Operator : RelationalOperator  Operator=>  OutDataTypeStr=boolean  RndMeth=Nearest
  Relational Operator1 : RelationalOperator  Operator=<  OutDataTypeStr=boolean  RndMeth=Nearest
  Relational Operator2 : RelationalOperator  Operator=<  OutDataTypeStr=boolean  RndMeth=Nearest
  Sum : Sum  Inputs=|+-
  Switch{,1..3} (4 alike) : Switch  Criteria=u2 > Threshold  Threshold=0.5
  Terminator : Terminator
  停止 : Constant  Value=drivmode_STOP
  加速 : Constant  Value=drivmode_ACC
  定常1 : Constant  Value=drivmode_CONST
  減速力行 : Constant  Value=drivmode_GensokuRikko
  減速回生 : Constant  Value=drivmode_GensokuKaisei
  wires:
  Switch/1 -> Terminator/1  "state_driving"
  target_v_VL_kmph/1 -> Relational Operator/1, Memory/1, Sum/1
  Relational Operator1/1 -> Switch1/2
  Constant4/1 -> Relational Operator1/2
  Relational Operator/1 -> Switch/2
  Constant/1 -> Relational Operator/2
  停止/1 -> Switch/3
  Sum/1 -> Relational Operator1/1, Relational Operator2/1
  減速回生/1 -> Switch2/1
  Switch3/1 -> Switch1/1
  Constant6/1 -> Relational Operator2/2
  Memory/1 -> Sum/2
  open_brake_per/1 -> Switch2/2
  減速力行/1 -> Switch2/3
  Relational Operator2/1 -> Switch3/2
  Switch2/1 -> Switch3/1
  定常1/1 -> Switch3/3
  加速/1 -> Switch1/3
  Switch1/1 -> Switch/1

== system METI_TRAMI_Thermal_ver01_Jmaab_2018b_Intg/Driver/Driver_TRAMI/Driver2/Caliculate_Opeining_Accel ==
  v_VL_PNT_kmph : Inport
  target_v_VL_kmph : Inport  Port=2
  pre_n_eng_rpm : Inport  Port=3
  pre_ratio_DCT : Inport  Port=4
  FB : Subsystem  mask{P_Gain=ACC_P_Gain, D_Gain=ACC_D_Gain, I_Gain=ACC_I_Gain}
      mask prompts: P_Gain "Pゲイン値"; D_Gain "Dゲイン値"; I_Gain "Iゲイン値"
  FF : Subsystem
  Guard_0_100 : Saturate  UpperLimit=ENG_CNT_Throttle_UL  LowerLimit=ENG_CNT_Throttle_LL
  Sum1 : Sum  Inputs=|-+
  Sum3 : Sum  Inputs=++|
  open_accel_per : Outport
  wires:
  Sum1/1 -> FB/1(delta_v_VL_kmph)
  v_VL_PNT_kmph/1 -> FF/1(v_VL_PNT_kmph), Sum1/1
  target_v_VL_kmph/1 -> FF/2(target_v_VL_kmph), Sum1/2
  Sum3/1 -> Guard_0_100/1
  pre_n_eng_rpm/1 -> FF/3(pre_n_eng_rpm)
  pre_ratio_DCT/1 -> FF/4(pre_ratio_DCT)
  FB/1(FB_open_accel_per) -> Sum3/1
  FF/1(FF_open_accel_per) -> Sum3/2
  Guard_0_100/1 -> open_accel_per/1  "open_accel_per"

== system METI_TRAMI_Thermal_ver01_Jmaab_2018b_Intg/Driver/Driver_TRAMI/Driver2/Caliculate_Opening_Brake ==
  v_VL_PNT_kmph : Inport
  target_v_VL_kmph : Inport  Port=2
  open_accel_per : Inport  Port=3
  Constant : Constant  Value=Driver_Brake_Const1
  Constant1 : Constant  Value=Driver_Brk_sh
  Constant2 : Constant  Value=Driver_Brake_Const3
  Constant3 : Constant  Value=0
  F2per : Gain  Gain=1/Brk_UL*100
  Logical Operator : Logic  AllPortsSameDT=off  OutDataTypeStr=boolean
  Memory : Memory
  Memory1 : Memory
  PGain : Gain  Gain=Brk_PGain
  PGain1 : Gain  Gain=Brk_PGain
  Relational Operator : RelationalOperator  OutDataTypeStr=boolean  RndMeth=Nearest
  Relational Operator1 : RelationalOperator  Operator=>  OutDataTypeStr=boolean  RndMeth=Nearest
  Saturation : Saturate  UpperLimit=Brk_UL  LowerLimit=Brk_LL
  Sum1 : Sum  Inputs=|-+
  Sum2 : Sum  Inputs=|+-
  Switch : Switch  Threshold=0.5
  Switch1 : Switch  Criteria=u2 > Threshold  Threshold=Driver_Brake_Switch_Const2
  open_brake_per : Outport
  wires:
  target_v_VL_kmph/1 -> Switch1/2, Sum1/2, Memory1/1, Sum2/1
  Sum1/1 -> PGain/1
  PGain/1 -> Saturation/1
  Constant/1 -> PGain1/1
  PGain1/1 -> Switch1/3
  open_accel_per/1 -> Memory/1
  Memory/1 -> Relational Operator1/1
  Memory1/1 -> Sum2/2
  Switch/1 -> F2per/1
  Sum2/1 -> Relational Operator/1
  Saturation/1 -> Switch1/1
  Switch1/1 -> Switch/3
  Constant2/1 -> Switch/1
  v_VL_PNT_kmph/1 -> Sum1/1
  Constant1/1 -> Relational Operator/2
  Constant3/1 -> Relational Operator1/2
  Relational Operator1/1 -> Logical Operator/2
  Relational Operator/1 -> Logical Operator/1
  Logical Operator/1 -> Switch/2
  F2per/1 -> open_brake_per/1  "open_brake_per"

== system METI_TRAMI_Thermal_ver01_Jmaab_2018b_Intg/Vehicle/ALT_PNT/Subsystem/I_alt_cal ==
  target_volt_ALT_V : Inport
  volt_BT_PNT_Lo_V : Inport  Port=2
  rpm_alt : Inport  Port=3
  Add : Sum
  Cal_I_alt_P_control : Subsystem
  Cal_I_alt_base : Subsystem
  Constant : Constant  Value=12
  Constant4 : Constant  Value=0
  Limit_Current_Max : Lookup_n-D  NumberOfTableDimensions=1  BreakpointsForDimension1=ALT_PNT_Alter_limit_Current_V_table_x_rpm  Table=ALT_PNT_Alter_limit_Current_V_table  ExtrapMethod=Clip  UseLastTableValue=on  RndMeth=Simplest  InputSameDT=on
  MinMax2 : MinMax  Function=max  Inputs=2
  Sum1 : Sum  Inputs=|+-
  Sum2 : Sum  Inputs=-+|
  電圧比較 : MinMax  Inputs=2
  I_alt : Outport
  wires:
  target_volt_ALT_V/1 -> Sum1/1, Sum2/2
  volt_BT_PNT_Lo_V/1 -> Sum2/1
  rpm_alt/1 -> Limit_Current_Max/1
  Constant4/1 -> MinMax2/2
  Limit_Current_Max/1 -> MinMax2/1  "I_limit_ALT"
  電圧比較/1 -> I_alt/1
  Add/1 -> 電圧比較/2
  Sum2/1 -> Cal_I_alt_P_control/1(V_delt_tgt)
  MinMax2/1 -> 電圧比較/1
  Constant/1 -> Sum1/2
  Sum1/1 -> Cal_I_alt_base/1(V_delt_tgt)
  Cal_I_alt_P_control/1(I_alt_base) -> Add/1
  Cal_I_alt_base/1(I_alt_base) -> Add/2

== system METI_TRAMI_Thermal_ver01_Jmaab_2018b_Intg/Vehicle/ALT_PNT/Subsystem/Torque_Guard ==
  current_ALT_PNT_A : Inport
  V_ALT_PNT : Inport  Port=2
  n_ROT_slavepulley12_rpm : Inport  Port=3
  ALT_GDCurrent : Inport  Port=4
  ALT_GDVolt : Inport  Port=5
  Caliculate_Axes_Torque1 : Lookup_n-D  NumberOfTableDimensions=3  BreakpointsForDimension1=ALT_PNT_Alter_trq_Nm_map_x_rpm  BreakpointsForDimension2=ALT_PNT_Alter_trq_Nm_map_y_Current_A  BreakpointsForDimension3=ALT_PNT_Alter_trq_Nm_map_z_Volt_tgt_V  Table=ALT_PNT_Alter_trq_Nm_map  RndMeth=Simplest  InputSameDT=on
  Caliculate_Axes_Torque2 : Lookup_n-D  NumberOfTableDimensions=3  BreakpointsForDimension1=ALT_PNT_Alter_trq_Nm_map_x_rpm  BreakpointsForDimension2=ALT_PNT_Alter_trq_Nm_map_y_Current_A  BreakpointsForDimension3=ALT_PNT_Alter_trq_Nm_map_z_Volt_tgt_V  Table=ALT_PNT_Alter_trq_Nm_map  RndMeth=Simplest  InputSameDT=on
  Constant3 : Constant  Value=ALT_PNT_trq_alter_output_LL_Nm
  MinMax : MinMax  Inputs=2
  MinMax1 : MinMax  Function=max  Inputs=2
  trq_trqsource : Outport
  wires:
  ALT_GDCurrent/1 -> Caliculate_Axes_Torque2/2
  Caliculate_Axes_Torque2/1 -> MinMax/2
  MinMax/1 -> MinMax1/1
  Caliculate_Axes_Torque1/1 -> MinMax/1
  Constant3/1 -> MinMax1/2
  ALT_GDVolt/1 -> Caliculate_Axes_Torque2/3
  MinMax1/1 -> trq_trqsource/1
  V_ALT_PNT/1 -> Caliculate_Axes_Torque1/3
  current_ALT_PNT_A/1 -> Caliculate_Axes_Torque1/2
  n_ROT_slavepulley12_rpm/1 -> Caliculate_Axes_Torque2/1, Caliculate_Axes_Torque1/1

== system METI_TRAMI_Thermal_ver01_Jmaab_2018b_Intg/Vehicle/BT_PNT_Lo/Cal_SOC/Subsystem4 ==
  In1 : Inport
  In2 : Inport  Port=2
  To Workspace : ToWorkspace  VariableName=SOC_LoBat  SampleTime=-1
      settings: Decimation=num_tws_mabiki
  To Workspace1 : ToWorkspace  VariableName=Asec_LoBat  SampleTime=-1
      settings: Decimation=num_tws_mabiki
  wires:
  In1/1 -> To Workspace/1
  In2/1 -> To Workspace1/1

== system METI_TRAMI_Thermal_ver01_Jmaab_2018b_Intg/Vehicle/CNT/ALT_CNT/ALT_Ctrl ==
  note: 【発電禁止条件】
      | 下記条件いずれかが成立時はオルタネータの発電を禁止する
      |   (2)エンジン停止中
      |   (3)エンジン始動中(下記エンジン回転数で判定)
      |      ene ≦ ALT_ON_RPM_HYS(1000[rpm])
      |                    ヒスあり(400[rpm])
  note: 【強制回生モード切替条件】
  note: 【回生モード切替条件】
      | 減速時FC中
  note: 例) 12[V]
  note: 例) 14[V]
  note: 例) 13.5[V]
  SOC_BT_PNT_Lo_PCT : Inport
  flag_fuelcut : Inport  Port=2
  flag_IdleStop : Inport  Port=3
  n_eng_rpm : Inport  Port=4
  Constant : Constant  Value=ALT_CNT_Alter_V_Kaisei_V
  Constant1 : Constant  Value=ALT_CNT_V_Battely_Kudo_V
  Constant2 : Constant  Value=ALT_CNT_flag_disable_kaisei
  Constant3 : Constant  Value=ALT_CNT_Alter_V_BASE_V
  Constant4 : Constant  Value=BT_PNT_Lo_SOC_MAX_lo_batt
  Logical Operator : Logic  Operator=OR  Inputs=3  AllPortsSameDT=off  OutDataTypeStr=boolean
  Logical Operator1 : Logic  AllPortsSameDT=off  OutDataTypeStr=boolean
  Logical Operator2 : Logic  Operator=NOT  AllPortsSameDT=off  OutDataTypeStr=boolean
  Relational Operator : RelationalOperator  OutDataTypeStr=boolean  RndMeth=Nearest
  Relay1 : Relay  OnSwitchValue=ALT_CNT_ALT_ON_RPM_HYS_rpm  OffSwitchValue=ALT_CNT_ALT_OFF_RPM_HYS_rpm  OnOutputValue=0  OffOutputValue=1
  Switch1 : Switch  Criteria=u2 > Threshold  Threshold=0.5
  Switch3 : Switch  Criteria=u2 > Threshold  Threshold=0.5
  target_volt_ALT_V : Outport
  wires:
  Switch3/1 -> target_volt_ALT_V/1  "target_volt_ALT_V"
  Constant3/1 -> Switch3/1
  Logical Operator2/1 -> Logical Operator1/2
  SOC_BT_PNT_Lo_PCT/1 -> Relational Operator/1
  Constant2/1 -> Switch3/2
  flag_fuelcut/1 -> Logical Operator1/1
  Relational Operator/1 -> Logical Operator/3
  Constant4/1 -> Relational Operator/2
  Logical Operator1/1 -> Switch1/2
  Logical Operator/1 -> Logical Operator2/1
  Constant/1 -> Switch1/1
  Relay1/1 -> Logical Operator/2
  Switch1/1 -> Switch3/3
  Constant1/1 -> Switch1/3
  flag_IdleStop/1 -> Logical Operator/1
  n_eng_rpm/1 -> Relay1/1

== system METI_TRAMI_Thermal_ver01_Jmaab_2018b_Intg/Vehicle/CNT/BK_CNT/BK_Ctrl ==
  open_brake_per_in : Inport
  v_VL_PNT_kmph_in : Inport  Port=2
  trq_BK_PNT_Nm_in : Inport  Port=3
  open_brake_per : Outport
  v_VL_PNT_kmph : Outport  Port=2
  trq_BK_PNT_Nm : Outport  Port=3
  wires:
  v_VL_PNT_kmph_in/1 -> v_VL_PNT_kmph/1
  trq_BK_PNT_Nm_in/1 -> trq_BK_PNT_Nm/1
  open_brake_per_in/1 -> open_brake_per/1

== system METI_TRAMI_Thermal_ver01_Jmaab_2018b_Intg/Vehicle/CNT/CAN/ALT_CNT ==
  note: ALT_Ctrl
  Pwtr_CAN : Inport
  Bus Creator2 : BusCreator  Inputs=3
  Bus Selector3 : BusSelector  OutputSignals=ENG_CNT_CAN_Tx
  Bus Selector4 : BusSelector  OutputSignals=flag_fuelcut,flag_IdleStop,n_eng_rpm
  tag scope: ALT_CNT_CAN_Rx=scoped
  wires:
  Bus Selector4/2 -> Bus Creator2/2  "<flag_IdleStop>"
  Bus Selector4/3 -> Bus Creator2/3  "<n_eng_rpm>"
  Pwtr_CAN/1 -> Bus Selector3/1
  Bus Creator2/1 -> [ALT_CNT_CAN_Rx]  "ALT_CNT_CAN_Rx"
  Bus Selector4/1 -> Bus Creator2/1  "<flag_fuelcut>"
  Bus Selector3/1 -> Bus Selector4/1  "<ENG_CNT_CAN_Tx>"

== system METI_TRAMI_Thermal_ver01_Jmaab_2018b_Intg/Vehicle/CNT/CAN/BK_CNT ==
  note: BK_Ctrl
  Pwtr_CAN : Inport
  Terminator : Terminator
  BK_CNT_CAN_Tx : Outport
  wires:
  [BK_CNT_CAN_Tx] -> BK_CNT_CAN_Tx/1
  Pwtr_CAN/1 -> Terminator/1

== system METI_TRAMI_Thermal_ver01_Jmaab_2018b_Intg/Vehicle/CNT/CAN/ENG_CNT ==
  note: ENG_Ctrl
  Pwtr_CAN : Inport
  Bus Creator3 : BusCreator  Inputs=2
  Bus Selector1 : BusSelector  OutputSignals=TM_CNT_CAN_Tx,BK_CNT_CAN_Tx
  Bus Selector2 : BusSelector  OutputSignals=flag_Lockup
  Bus Selector3 : BusSelector  OutputSignals=v_VL_PNT_kmph
  ENG_CNT_CAN_Tx : Outport
  tag scope: ENG_CNT_CAN_Rx=scoped
  wires:
  Bus Creator3/1 -> [ENG_CNT_CAN_Rx]  "ENG_CNT_CAN_Rx"
  Bus Selector1/1 -> Bus Selector2/1  "<TM_CNT_CAN_Tx>"
  Bus Selector2/1 -> Bus Creator3/1  "<flag_Lockup>"
  Pwtr_CAN/1 -> Bus Selector1/1
  [ENG_CNT_CAN_Tx] -> ENG_CNT_CAN_Tx/1
  Bus Selector1/2 -> Bus Selector3/1  "<BK_CNT_CAN_Tx>"
  Bus Selector3/1 -> Bus Creator3/2  "<v_VL_PNT_kmph>"

== system METI_TRAMI_Thermal_ver01_Jmaab_2018b_Intg/Vehicle/CNT/CAN/Pwtr_CAN ==
  note: 通信遅れ無し
  ENG_CNT_CAN_Tx : Inport
  TM_CNT_CAN_Tx : Inport  Port=2
  BK_CNT_CAN_Tx : Inport  Port=3
  Bus Creator8 : BusCreator  Inputs=3
  Unit Delay : UnitDelay  SampleTime=-1
  Pwtr_CAN : Outport
  wires:
  ENG_CNT_CAN_Tx/1 -> Bus Creator8/1
  TM_CNT_CAN_Tx/1 -> Bus Creator8/2
  Unit Delay/1 -> Pwtr_CAN/1  "Pwtr_CAN"
  Bus Creator8/1 -> Unit Delay/1
  BK_CNT_CAN_Tx/1 -> Bus Creator8/3

== system METI_TRAMI_Thermal_ver01_Jmaab_2018b_Intg/Vehicle/CNT/CAN/TM_CNT ==
  note: TM_Ctrl
  Pwtr_CAN : Inport
  Bus Creator4 : BusCreator  Inputs=5
  Bus Selector3 : BusSelector  OutputSignals=v_VL_PNT_kmph,trq_BK_PNT_Nm
  Bus Selector5 : BusSelector  OutputSignals=ENG_CNT_CAN_Tx,BK_CNT_CAN_Tx
  Bus Selector6 : BusSelector  OutputSignals=open_throttle_per,T_ENGTH_PNT_Coolant_degC,IdleSpeed_Target
  TM_CNT_CAN_Tx : Outport
  tag scope: TM_CNT_CAN_Rx=scoped
  wires:
  Bus Selector5/1 -> Bus Selector6/1  "<ENG_CNT_CAN_Tx>"
  Bus Selector6/1 -> Bus Creator4/1  "<open_throttle_per>"
  Pwtr_CAN/1 -> Bus Selector5/1
  Bus Creator4/1 -> [TM_CNT_CAN_Rx]  "TM_CNT_CAN_Rx"
  [TM_CNT_CAN_Tx] -> TM_CNT_CAN_Tx/1
  Bus Selector6/2 -> Bus Creator4/2  "<T_ENGTH_PNT_Coolant_degC>"
  Bus Selector5/2 -> Bus Selector3/1  "<BK_CNT_CAN_Tx>"
  Bus Selector3/1 -> Bus Creator4/4  "<v_VL_PNT_kmph>"
  Bus Selector3/2 -> Bus Creator4/5  "<trq_BK_PNT_Nm>"
  Bus Selector6/3 -> Bus Creator4/3  "<IdleSpeed_Target>"

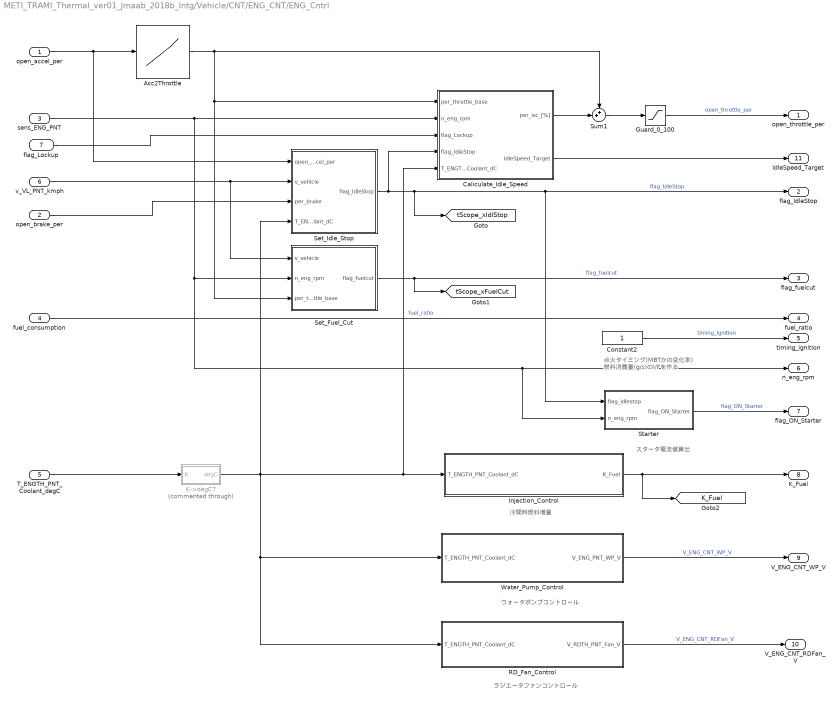
== system METI_TRAMI_Thermal_ver01_Jmaab_2018b_Intg/Vehicle/CNT/ENG_CNT/ENG_Cntrl ==
  note: ラジエータファンコントロール
  note: ウォータポンプコントロール
  note: 冷間時燃料増量
  note: スタータ電流値算出
  note: 点火タイミング(MBTかの変化率)
      | 燃料消費量(g/s)のI/Fを作る
  open_accel_per : Inport
  open_brake_per : Inport  Port=2
  sens_ENG_PNT : Inport  Port=3
  fuel_consumption : Inport  Port=4
  T_ENGTH_PNT_Coolant_degC : Inport  Port=5
  v_VL_PNT_kmph : Inport  Port=6
  flag_Lockup : Inport  Port=7
  Acc2Throttle : Lookup_n-D  NumberOfTableDimensions=1  BreakpointsForDimension1=[ENG_CNT_Accel_LL:ENG_CNT_Accel_UL]  Table=[ENG_CNT_Throttle_LL:ENG_CNT_Throttle_UL]  RndMeth=Simplest  InputSameDT=on
  Caliculate_Idle_Speed : Subsystem
  Constant2 : Constant
  Guard_0_100 : Saturate  UpperLimit=ENG_CNT_Throttle_UL  LowerLimit=ENG_CNT_Throttle_LL
  Injection_Control : Subsystem
  K->degC7 : Subsystem  Commented=through
  RD_Fan_Control : Subsystem
  Set_Fuel_Cut : Subsystem
  Set_Idle_Stop : Subsystem
  Starter : Subsystem
  Sum1 : Sum  Inputs=++|
  Water_Pump_Control : Subsystem
  open_throttle_per : Outport
  flag_IdleStop : Outport  Port=2
  flag_fuelcut : Outport  Port=3
  fuel_ratio : Outport  Port=4
  timing_ignition : Outport  Port=5
  n_eng_rpm : Outport  Port=6
  flag_ON_Starter : Outport  Port=7
  K_Fuel : Outport  Port=8
  V_ENG_CNT_WP_V : Outport  Port=9
  V_ENG_CNT_RDFan_V : Outport  Port=10
  IdleSpeed_Target : Outport  Port=11
  tag scope: K_Fuel=global, tScope_xFuelCut=global, tScope_xIdlStop=global
  wires:
  Caliculate_Idle_Speed/2(IdleSpeed_Target) -> IdleSpeed_Target/1
  K->degC7/1(degC) -> Caliculate_Idle_Speed/5(T_ENGTH_PNT_Coolant_dC), Injection_Control/1(T_ENGTH_PNT_Coolant_dC), Set_Idle_Stop/4(T_ENGTH_PNT_Coolant_dC), Water_Pump_Control/1(T_ENGTH_PNT_Coolant_dC), RD_Fan_Control/1(T_ENGTH_PNT_Coolant_dC)
  RD_Fan_Control/1(V_RDTH_PNT_Fan_V) -> V_ENG_CNT_RDFan_V/1  "V_ENG_CNT_RDFan_V"
  Injection_Control/1(K_Fuel) -> K_Fuel/1, [K_Fuel]
  T_ENGTH_PNT_Coolant_degC/1 -> K->degC7/1(K)
  Water_Pump_Control/1(V_ENG_PNT_WP_V) -> V_ENG_CNT_WP_V/1  "V_ENG_CNT_WP_V"
  flag_Lockup/1 -> Caliculate_Idle_Speed/3(flag_Lockup)
  Starter/1(flag_ON_Starter) -> flag_ON_Starter/1  "flag_ON_Starter"
  v_VL_PNT_kmph/1 -> Set_Idle_Stop/2(v_vehicle), Set_Fuel_Cut/1(v_vehicle)
  open_accel_per/1 -> Set_Idle_Stop/1(open_accel_per), Acc2Throttle/1
  open_brake_per/1 -> Set_Idle_Stop/3(per_brake)
  sens_ENG_PNT/1 -> Starter/2(n_eng_rpm), n_eng_rpm/1, Set_Fuel_Cut/2(n_eng_rpm), Caliculate_Idle_Speed/2(n_eng_rpm)
  Guard_0_100/1 -> open_throttle_per/1  "open_throttle_per"
  Set_Fuel_Cut/1(flag_fuelcut) -> [tScope_xFuelCut], flag_fuelcut/1  "flag_fuelcut"
  Constant2/1 -> timing_ignition/1  "timing_ignition"
  fuel_consumption/1 -> fuel_ratio/1  "fuel_ratio"
  Acc2Throttle/1 -> Set_Fuel_Cut/3(per_throttle_base), Caliculate_Idle_Speed/1(per_throttle_base), Sum1/1
  Sum1/1 -> Guard_0_100/1
  Caliculate_Idle_Speed/1(per_isc_[%]) -> Sum1/2
  Set_Idle_Stop/1(flag_IdleStop) -> Caliculate_Idle_Speed/4(flag_IdleStop), flag_IdleStop/1, Starter/1(flag_idlestop), [tScope_xIdlStop]  "flag_IdleStop"

== system METI_TRAMI_Thermal_ver01_Jmaab_2018b_Intg/Vehicle/CNT/TM_CNT/TM_CNT ==
  "sensor_TM_PNT " : Inport
  "TM_CNT_CAN_Rx " : Inport  Port=2
  TM_CNT : Subsystem  TreatAsAtomicUnit=on  VariantControl=VarObj_METI_Subsys
      settings: AttributesFormatString="<AtomicUnit =  %<TreatAsAtomicUnit>>"
  TM_CNT1 : ModelReference  ModelNameDialog=METI_TM_CNT  SimulationMode=Normal  VariantControl=VarObj_METI_Mref  ModelReferenceVersion=1.420
  TM_CNT2 : ModelReference  ModelNameDialog=TRAMI_TM_CNT  SimulationMode=Normal  VariantControl=VarObj_TRAMI_Mref  ModelReferenceVersion=1.399
  " TM_CNT_out" : Outport
  " TM_CNT_CAN_Tx" : Outport  Port=2
  " TM_CNT_Info" : Outport  Port=3

== system METI_TRAMI_Thermal_ver01_Jmaab_2018b_Intg/Vehicle/ENG_PNT/ENG_Plant/Cal_FuelComsunption ==
  w_ENG_PNT_radps : Inport
  trq_ENG : Inport  Port=2
  flag_fuelcut : Inport  Port=3
  flag_IdleStop : Inport  Port=4
  timing_ignition : Inport  Port=5
  K_Fuel : Inport  Port=6
  1-D Lookup Table1 : Lookup_n-D  NumberOfTableDimensions=1  BreakpointsForDimension1=ENG_PNT_trq_fluc_Nm_table_x_spk_tim  Table=ENG_PNT_trq_fluc_Nm_table  RndMeth=Simplest  InputSameDT=on
  Map_FuelRate : Lookup_n-D  BreakpointsForDimension1=ENG_PNT_FuelCon_gps_map_y_trq_Nm  BreakpointsForDimension2=ENG_PNT_FuelCon_gps_map_x_pri_rpm  Table=ENG_PNT_FuelCon_gps_map  RndMeth=Simplest  InputSameDT=on
  Not_cal1 : Subsystem
  Not_cal2 : Subsystem
  Product : Product  Inputs=4  RndMeth=Zero
  Product1 : Product  Inputs=*/  RndMeth=Zero
  radpsec2rpm : Gain  Gain=radpsec2rpm
  FuelConsumption : Outport
  wires:
  trq_ENG/1 -> Product1/1
  radpsec2rpm/1 -> Map_FuelRate/2
  w_ENG_PNT_radps/1 -> radpsec2rpm/1
  Product/1 -> FuelConsumption/1
  Not_cal2/1(Out1) -> Product/3
  Not_cal1/1(Out1) -> Product/2
  flag_fuelcut/1 -> Not_cal1/1(In1)
  flag_IdleStop/1 -> Not_cal2/1(In1)
  timing_ignition/1 -> 1-D Lookup Table1/1
  1-D Lookup Table1/1 -> Product1/2
  Product1/1 -> Map_FuelRate/1
  Map_FuelRate/1 -> Product/1
  K_Fuel/1 -> Product/4

== system METI_TRAMI_Thermal_ver01_Jmaab_2018b_Intg/Vehicle/ENG_PNT/ENG_Plant/Cal_trq_ENG_jiku ==
  note: エンジン軸トルクマップ
  open_throttle_per : Inport
  flag_fuelcut : Inport  Port=2
  flag_IdleStop : Inport  Port=3
  timing_ignition : Inport  Port=4
  w_ENG_PNT_radps : Inport  Port=5
  1-D Lookup Table : Lookup_n-D  NumberOfTableDimensions=1  BreakpointsForDimension1=ENG_PNT_trq_fluc_Nm_table_x_spk_tim  Table=ENG_PNT_trq_fluc_Nm_table  RndMeth=Simplest  InputSameDT=on
  2-D Lookup Table : Lookup_n-D  BreakpointsForDimension1=ENG_PNT_trq_Nm_map_y_throttle  BreakpointsForDimension2=ENG_PNT_trq_Nm_map_x_rpm  Table=ENG_PNT_trq_Nm_map  ExtrapMethod=Clip  UseLastTableValue=on  RndMeth=Simplest  InputSameDT=on
  Model Info : simulink/Model-Wide Utilities/Model Info  Frame=on  DisplayStringWithTags=|  HorizontalTextAlignment=Left  LeftAlignmentValue=0.02
      | 【注記】
      | ・燃料カット時はスロットル開度を0としてエンジンフリクションを付加
      | ・点火タイミングによるトルク変動を想定
      | ・エンジン軸トルクマップの使用
  Not_cal : Subsystem
  Not_cal1 : Subsystem
  Product : Product  RndMeth=Zero
  Product1 : Product  RndMeth=Zero
  Product2 : Product  RndMeth=Zero
  Saturation : Saturate  UpperLimit=ENG_CNT_Throttle_UL  LowerLimit=ENG_CNT_Throttle_LL
  radpsec2rpm : Gain  Gain=radpsec2rpm
  trq_ENG_PNT_Nm : Outport
  wires:
  w_ENG_PNT_radps/1 -> radpsec2rpm/1
  2-D Lookup Table/1 -> Product1/1
  open_throttle_per/1 -> Product/1
  Saturation/1 -> 2-D Lookup Table/1
  radpsec2rpm/1 -> 2-D Lookup Table/2
  timing_ignition/1 -> 1-D Lookup Table/1
  1-D Lookup Table/1 -> Product1/2
  Product/1 -> Saturation/1
  Product2/1 -> Product/2
  flag_fuelcut/1 -> Not_cal/1(In1)
  Not_cal/1(Out1) -> Product2/1
  flag_IdleStop/1 -> Not_cal1/1(In1)
  Not_cal1/1(Out1) -> Product2/2
  Product1/1 -> trq_ENG_PNT_Nm/1  "trq_ENG_PNT_Nm"

== system METI_TRAMI_Thermal_ver01_Jmaab_2018b_Intg/Vehicle/ENG_PNT/ENG_Plant/Coldstart_Additional_friction_calc2 ==
  note: スロットル開度0の時の
      | 軸トルクを読み出し
  T_ENGOil_degC : Inport
  w_ENG_PNT_radps : Inport  Port=2
  1-D Lookup Table : Lookup_n-D  NumberOfTableDimensions=1  BreakpointsForDimension1=ENG_PNT_Cold_friction_gain_x_T_ENGOil  Table=ENG_PNT_Cold_friction_gain  InternalRulePriority=Speed  RndMeth=Simplest  InputSameDT=on
  2-D Lookup Table : Lookup_n-D  BreakpointsForDimension1=ENG_PNT_trq_Nm_map_y_throttle  BreakpointsForDimension2=ENG_PNT_trq_Nm_map_x_rpm  Table=ENG_PNT_trq_Nm_map  ExtrapMethod=Clip  UseLastTableValue=on  RndMeth=Simplest  InputSameDT=on
  Add : Sum  Inputs=+-
  Constant1 : Constant  Value=0
  Product : Product
  radpsec2rpm : Gain  Gain=radpsec2rpm
  Additional_friction : Outport
  wires:
  T_ENGOil_degC/1 -> 1-D Lookup Table/1
  w_ENG_PNT_radps/1 -> radpsec2rpm/1
  radpsec2rpm/1 -> 2-D Lookup Table/2
  Constant1/1 -> 2-D Lookup Table/1
  2-D Lookup Table/1 -> Add/2, Product/2
  1-D Lookup Table/1 -> Product/1
  Add/1 -> Additional_friction/1
  Product/1 -> Add/1

== system METI_TRAMI_Thermal_ver01_Jmaab_2018b_Intg/Vehicle/ENG_PNT/ENG_Plant/Coldstart_Heat_flux_gain_calc ==
  T_ENGOil_degC : Inport
  1-D Lookup Table : Lookup_n-D  NumberOfTableDimensions=1  BreakpointsForDimension1=ENG_PNT_Heatflux2ENGOil_gain_x_T_ENGOil  Table=ENG_PNT_Heatflux2ENGOil_gain  InternalRulePriority=Speed  RndMeth=Simplest  InputSameDT=on
  Heat_flux_gain : Outport
  wires:
  T_ENGOil_degC/1 -> 1-D Lookup Table/1
  1-D Lookup Table/1 -> Heat_flux_gain/1

== system METI_TRAMI_Thermal_ver01_Jmaab_2018b_Intg/Vehicle/ENG_PNT/ENG_Plant/Coldstart_Heat_flux_gain_calc1 ==
  T_ENG_Cylinder_Head_degC : Inport
  1-D Lookup Table : Lookup_n-D  NumberOfTableDimensions=1  BreakpointsForDimension1=ENG_PNT_Heatflux2Cylinder_Head_gain_x_T_Coolant  Table=ENG_PNT_Heatflux2Cylinder_Head_gain  InternalRulePriority=Speed  RndMeth=Simplest  InputSameDT=on
  Heat_flux_gain : Outport
  wires:
  T_ENG_Cylinder_Head_degC/1 -> 1-D Lookup Table/1
  1-D Lookup Table/1 -> Heat_flux_gain/1

== system METI_TRAMI_Thermal_ver01_Jmaab_2018b_Intg/Vehicle/ENG_PNT/ENG_Plant/K->degC1 ==
  K : Inport
  Constant2 : Constant  Value=K2degC
  Sum : Sum  Inputs=++|
  degC : Outport
  wires:
  K/1 -> Sum/2
  Constant2/1 -> Sum/1
  Sum/1 -> degC/1

== system METI_TRAMI_Thermal_ver01_Jmaab_2018b_Intg/Vehicle/ENG_PNT/ENG_Plant/K->degC6 ==
  K : Inport
  Constant2 : Constant  Value=K2degC
  Sum : Sum  Inputs=++|
  degC : Outport
  wires:
  K/1 -> Sum/2
  Constant2/1 -> Sum/1
  Sum/1 -> degC/1

== system METI_TRAMI_Thermal_ver01_Jmaab_2018b_Intg/Vehicle/PTTH/ATM_PNT/degC->K ==
  degC : Inport
  Constant2 : Constant  Value=degC2K
  Sum : Sum  Inputs=++|
  K : Outport
  wires:
  degC/1 -> Sum/2
  Constant2/1 -> Sum/1
  Sum/1 -> K/1

== system METI_TRAMI_Thermal_ver01_Jmaab_2018b_Intg/Vehicle/PTTH/ATM_PNT/degC->K1 ==
  degC : Inport
  Constant2 : Constant  Value=degC2K
  Sum : Sum  Inputs=++|
  K : Outport
  wires:
  Sum/1 -> K/1
  Constant2/1 -> Sum/1
  degC/1 -> Sum/2

== system METI_TRAMI_Thermal_ver01_Jmaab_2018b_Intg/Vehicle/PTTH/ATM_PNT/degC->K2 ==
  degC : Inport
  Constant2 : Constant  Value=degC2K
  Sum : Sum  Inputs=++|
  K : Outport
  wires:
  degC/1 -> Sum/2
  Constant2/1 -> Sum/1
  Sum/1 -> K/1

== system METI_TRAMI_Thermal_ver01_Jmaab_2018b_Intg/Vehicle/PTTH/ATM_PNT/degC->K3 ==
  degC : Inport
  Constant2 : Constant  Value=degC2K
  Sum : Sum  Inputs=++|
  K : Outport
  wires:
  Sum/1 -> K/1
  Constant2/1 -> Sum/1
  degC/1 -> Sum/2
